simulink model "High_level_control_system_temporary_change"  (R2021b)
settings: Solver=VariableStepAuto  StartTime=0.0  StopTime=10.0  RelTol=1e-3
settings Model: Creator=louis  LastModifiedBy=louis

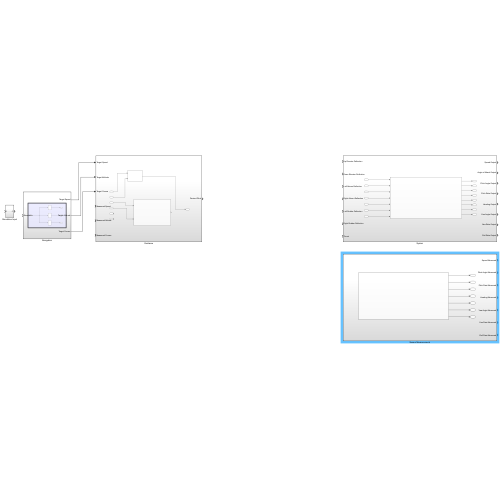
[thumbnail: Simulink's stored preview of the top-level diagram]
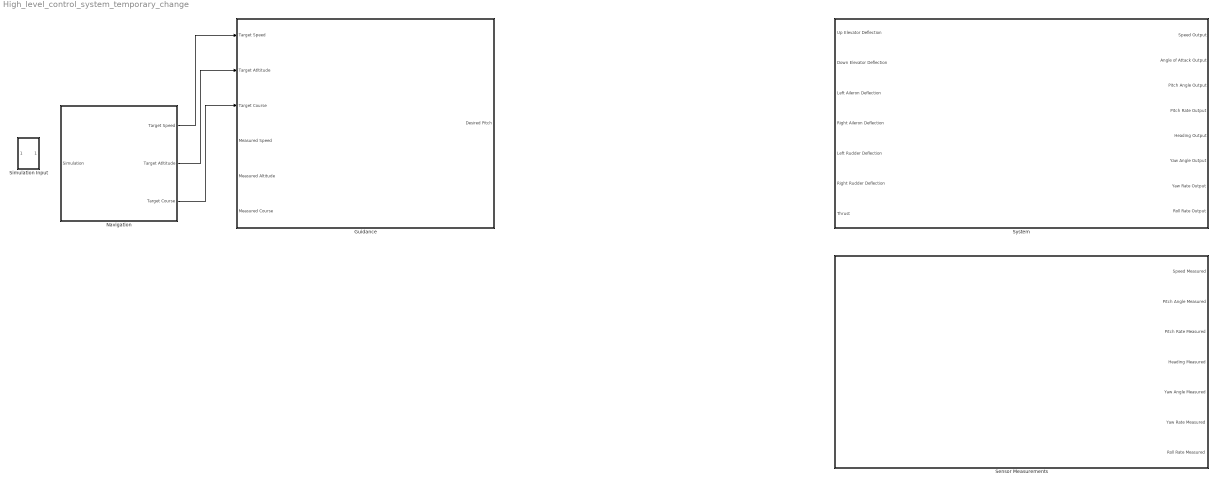
== system High_level_control_system_temporary_change ==
  Guidance : Subsystem
  Navigation : Subsystem
  Sensor Measurements : Subsystem
  Simulation Input : Subsystem
  System : Subsystem
  wires:
  Navigation/1(Target Speed) -> Guidance/1(Target Speed)
  Navigation/2(Target Atltitude) -> Guidance/2(Target Atltitude)
  Navigation/3(Target Course) -> Guidance/3(Target Course)

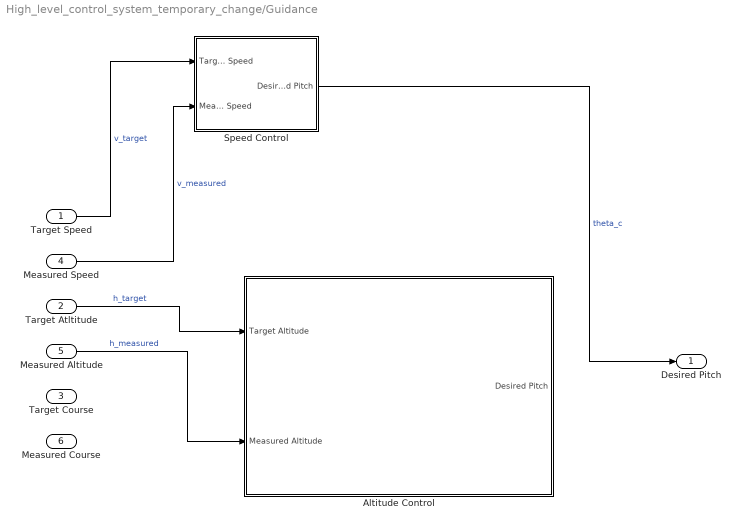
== system High_level_control_system_temporary_change/Guidance ==
  Target Speed : Inport
  Target Atltitude : Inport  Port=2
  Target Course : Inport  Port=3
  Measured Speed : Inport  Port=4
  Measured Altitude : Inport  Port=5
  Measured Course : Inport  Port=6
  Altitude Control : Subsystem
  Speed Control : Subsystem
  Desired Pitch : Outport
  wires:
  Target Speed/1 -> Speed Control/1(Target Speed)  "v_target"
  Measured Speed/1 -> Speed Control/2(Measured Speed)  "v_measured"
  Speed Control/1(Desired Pitch) -> Desired Pitch/1  "theta_c"
  Target Atltitude/1 -> Altitude Control/1(Target Altitude)  "h_target"
  Measured Altitude/1 -> Altitude Control/2(Measured Altitude)  "h_measured"

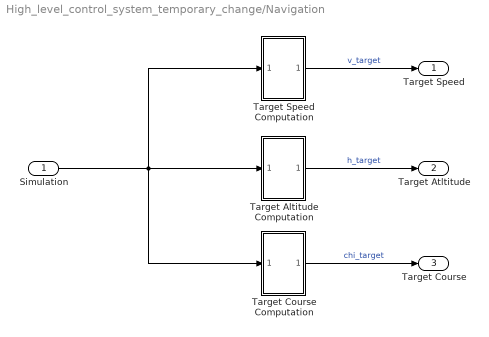
== system High_level_control_system_temporary_change/Navigation ==
  Simulation : Inport
  Target Altitude Computation : Subsystem
  Target Course Computation : Subsystem
  Target Speed Computation : Subsystem
  Target Speed : Outport
  Target Atltitude : Outport  Port=2
  Target Course : Outport  Port=3
  wires:
  Simulation/1 -> Target Speed Computation/1(In1), Target Altitude Computation/1(In1), Target Course Computation/1(In1)
  Target Speed Computation/1(Out1) -> Target Speed/1  "v_target"
  Target Altitude Computation/1(Out1) -> Target Atltitude/1  "h_target"
  Target Course Computation/1(Out1) -> Target Course/1  "chi_target"

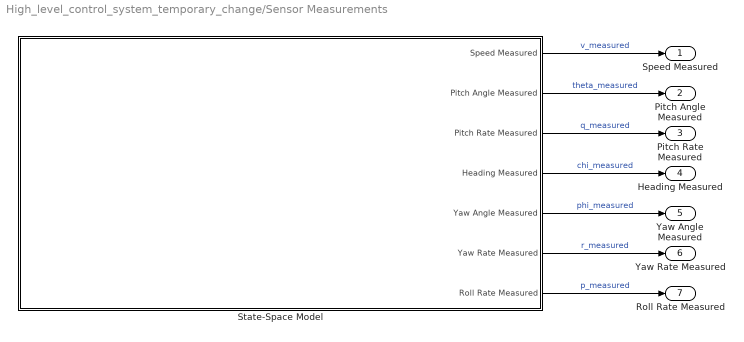
== system High_level_control_system_temporary_change/Sensor Measurements ==
  State-Space Model : Subsystem
  Speed Measured : Outport
  Pitch Angle Measured : Outport  Port=2
  Pitch Rate Measured : Outport  Port=3
  Heading Measured : Outport  Port=4
  Yaw Angle Measured : Outport  Port=5
  Yaw Rate Measured : Outport  Port=6
  Roll Rate Measured : Outport  Port=7
  wires:
  State-Space Model/7(Roll Rate Measured) -> Roll Rate Measured/1  "p_measured"
  State-Space Model/6(Yaw Rate Measured) -> Yaw Rate Measured/1  "r_measured"
  State-Space Model/5(Yaw Angle Measured) -> Yaw Angle Measured/1  "phi_measured"
  State-Space Model/2(Pitch Angle Measured) -> Pitch Angle Measured/1  "theta_measured"
  State-Space Model/3(Pitch Rate Measured) -> Pitch Rate Measured/1  "q_measured"
  State-Space Model/1(Speed Measured) -> Speed Measured/1  "v_measured"
  State-Space Model/4(Heading Measured) -> Heading Measured/1  "chi_measured"

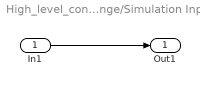
== system High_level_control_system_temporary_change/Simulation Input ==
  In1 : Inport
  Out1 : Outport
  wires:
  In1/1 -> Out1/1

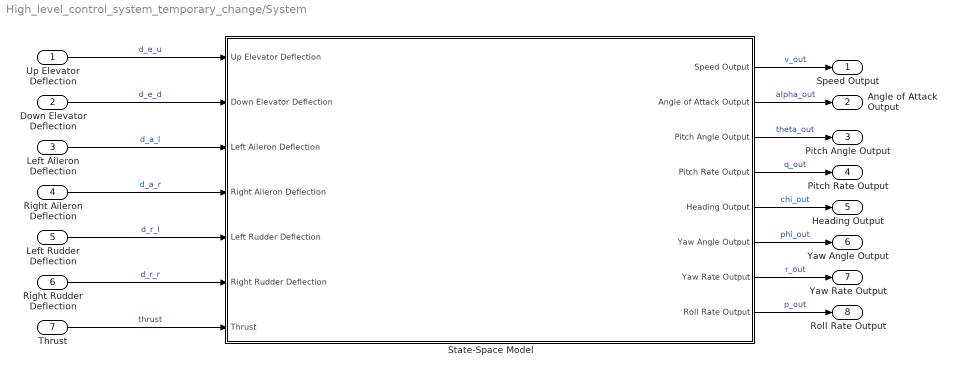
== system High_level_control_system_temporary_change/System ==
  Up Elevator Deflection : Inport
  Down Elevator Deflection : Inport  Port=2
  Left Aileron Deflection : Inport  Port=3
  Right Aileron Deflection : Inport  Port=4
  Left Rudder Deflection : Inport  Port=5
  Right Rudder Deflection : Inport  Port=6
  Thrust : Inport  Port=7
  State-Space Model : Subsystem
  Speed Output : Outport
  Angle of Attack Output : Outport  Port=2
  Pitch Angle Output : Outport  Port=3
  Pitch Rate Output : Outport  Port=4
  Heading Output : Outport  Port=5
  Yaw Angle Output : Outport  Port=6
  Yaw Rate Output : Outport  Port=7
  Roll Rate Output : Outport  Port=8
  wires:
  Up Elevator Deflection/1 -> State-Space Model/1(Up Elevator Deflection)  "d_e_u"
  Left Rudder Deflection/1 -> State-Space Model/5(Left Rudder Deflection)  "d_r_l"
  Left Aileron Deflection/1 -> State-Space Model/3(Left Aileron Deflection)  "d_a_l"
  Right Rudder Deflection/1 -> State-Space Model/6(Right Rudder Deflection)  "d_r_r"
  Right Aileron Deflection/1 -> State-Space Model/4(Right Aileron Deflection)  "d_a_r"
  Thrust/1 -> State-Space Model/7(Thrust)  "thrust"
  State-Space Model/8(Roll Rate Output) -> Roll Rate Output/1  "p_out"
  State-Space Model/1(Speed Output) -> Speed Output/1  "v_out"
  State-Space Model/5(Heading Output) -> Heading Output/1  "chi_out"
  State-Space Model/3(Pitch Angle Output) -> Pitch Angle Output/1  "theta_out"
  State-Space Model/2(Angle of Attack Output) -> Angle of Attack Output/1  "alpha_out"
  State-Space Model/4(Pitch Rate Output) -> Pitch Rate Output/1  "q_out"
  State-Space Model/6(Yaw Angle Output) -> Yaw Angle Output/1  "phi_out"
  State-Space Model/7(Yaw Rate Output) -> Yaw Rate Output/1  "r_out"
  Down Elevator Deflection/1 -> State-Space Model/2(Down Elevator Deflection)  "d_e_d"

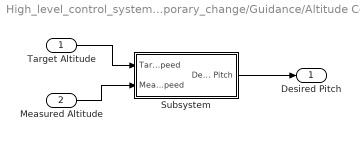
== system High_level_control_system_temporary_change/Guidance/Altitude Control ==
  Target Altitude : Inport
  Measured Altitude : Inport  Port=2
  Subsystem : Subsystem
  Desired Pitch : Outport
  wires:
  Target Altitude/1 -> Subsystem/1(Target Speed)
  Measured Altitude/1 -> Subsystem/2(Measured Speed)
  Subsystem/1(Desired Pitch) -> Desired Pitch/1

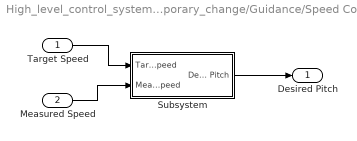
== system High_level_control_system_temporary_change/Guidance/Speed Control ==
  Target Speed : Inport
  Measured Speed : Inport  Port=2
  Subsystem : Subsystem
  Desired Pitch : Outport
  wires:
  Target Speed/1 -> Subsystem/1(Target Speed)
  Measured Speed/1 -> Subsystem/2(Measured Speed)
  Subsystem/1(Desired Pitch) -> Desired Pitch/1

== system High_level_control_system_temporary_change/Navigation/Target Altitude Computation ==
  In1 : Inport
  Out1 : Outport
  wires:
  In1/1 -> Out1/1

== system High_level_control_system_temporary_change/Navigation/Target Course Computation ==
  In1 : Inport
  Out1 : Outport
  wires:
  In1/1 -> Out1/1

== system High_level_control_system_temporary_change/Navigation/Target Speed Computation ==
  In1 : Inport
  Out1 : Outport
  wires:
  In1/1 -> Out1/1

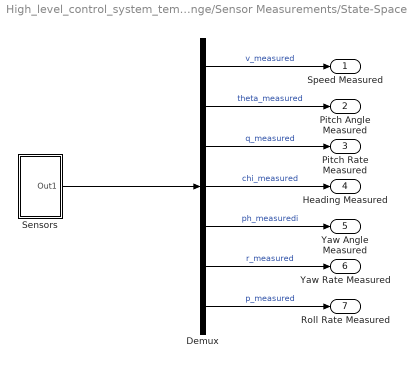
== system High_level_control_system_temporary_change/Sensor Measurements/State-Space Model ==
  Demux : Demux  Outputs=7
  Sensors : Subsystem
  Speed Measured : Outport
  Pitch Angle Measured : Outport  Port=2
  Pitch Rate Measured : Outport  Port=3
  Heading Measured : Outport  Port=4
  Yaw Angle Measured : Outport  Port=5
  Yaw Rate Measured : Outport  Port=6
  Roll Rate Measured : Outport  Port=7
  wires:
  Demux/7 -> Roll Rate Measured/1  "p_measured"
  Demux/3 -> Pitch Rate Measured/1  "q_measured"
  Demux/5 -> Yaw Angle Measured/1  "ph_measuredi"
  Demux/6 -> Yaw Rate Measured/1  "r_measured"
  Demux/1 -> Speed Measured/1  "v_measured"
  Demux/4 -> Heading Measured/1  "chi_measured"
  Demux/2 -> Pitch Angle Measured/1  "theta_measured"
  Sensors/1(Out1) -> Demux/1

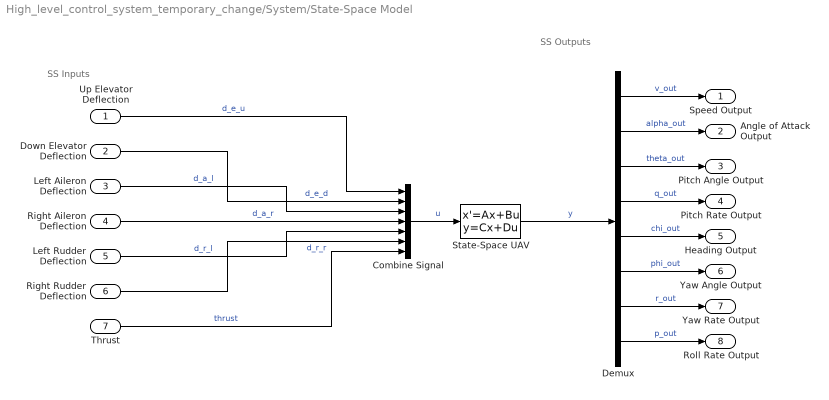
== system High_level_control_system_temporary_change/System/State-Space Model ==
  note: SS Outputs
  note: SS Inputs
  Up Elevator Deflection : Inport
  Down Elevator Deflection : Inport  Port=2
  Left Aileron Deflection : Inport  Port=3
  Right Aileron Deflection : Inport  Port=4
  Left Rudder Deflection : Inport  Port=5
  Right Rudder Deflection : Inport  Port=6
  Thrust : Inport  Port=7
  Combine Signal : Concatenate  NumInputs=7
  Demux : Demux  Outputs=8
  State-Space UAV : StateSpace  InitialCondition=0
  Speed Output : Outport
  Angle of Attack Output : Outport  Port=2
  Pitch Angle Output : Outport  Port=3
  Pitch Rate Output : Outport  Port=4
  Heading Output : Outport  Port=5
  Yaw Angle Output : Outport  Port=6
  Yaw Rate Output : Outport  Port=7
  Roll Rate Output : Outport  Port=8
  wires:
  Up Elevator Deflection/1 -> Combine Signal/1  "d_e_u"
  Left Aileron Deflection/1 -> Combine Signal/3  "d_a_l"
  Right Aileron Deflection/1 -> Combine Signal/4  "d_a_r"
  Left Rudder Deflection/1 -> Combine Signal/5  "d_r_l"
  Right Rudder Deflection/1 -> Combine Signal/6  "d_r_r"
  Thrust/1 -> Combine Signal/7  "thrust"
  Combine Signal/1 -> State-Space UAV/1  "u"
  State-Space UAV/1 -> Demux/1  "y"
  Demux/1 -> Speed Output/1  "v_out"
  Demux/2 -> Angle of Attack Output/1  "alpha_out"
  Demux/3 -> Pitch Angle Output/1  "theta_out"
  Demux/4 -> Pitch Rate Output/1  "q_out"
  Demux/5 -> Heading Output/1  "chi_out"
  Demux/6 -> Yaw Angle Output/1  "phi_out"
  Demux/7 -> Yaw Rate Output/1  "r_out"
  Demux/8 -> Roll Rate Output/1  "p_out"
  Down Elevator Deflection/1 -> Combine Signal/2  "d_e_d"

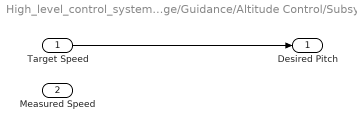
== system High_level_control_system_temporary_change/Guidance/Altitude Control/Subsystem ==
  Target Speed : Inport
  Measured Speed : Inport  Port=2
  Desired Pitch : Outport
  wires:
  Target Speed/1 -> Desired Pitch/1

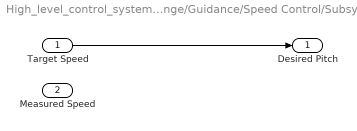
== system High_level_control_system_temporary_change/Guidance/Speed Control/Subsystem ==
  Target Speed : Inport
  Measured Speed : Inport  Port=2
  Desired Pitch : Outport
  wires:
  Target Speed/1 -> Desired Pitch/1

== system High_level_control_system_temporary_change/Sensor Measurements/State-Space Model/Sensors ==
  note: Sensors
  Out1 : Outport
